simulink model "parent_model"  (R2024a)
settings: Solver=VariableStepAuto  StartTime=0.0  StopTime=50  RelTol=1e-3
libraries: aerolibutil x3, sharedtransform x1
settings Model: Creator=aryam  LastModifiedBy=ashis
settings RTWCC: GPUComputeCapability=3.5

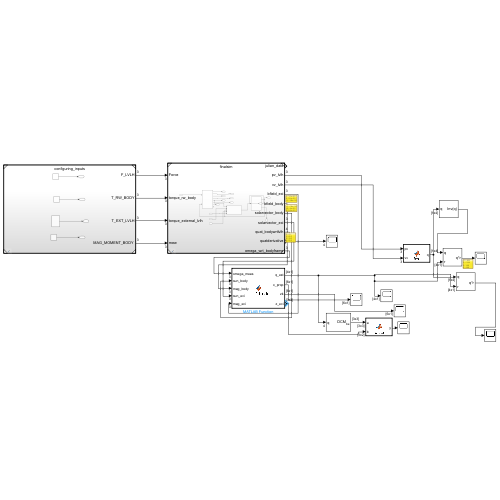
[thumbnail: Simulink's stored preview of the top-level diagram]
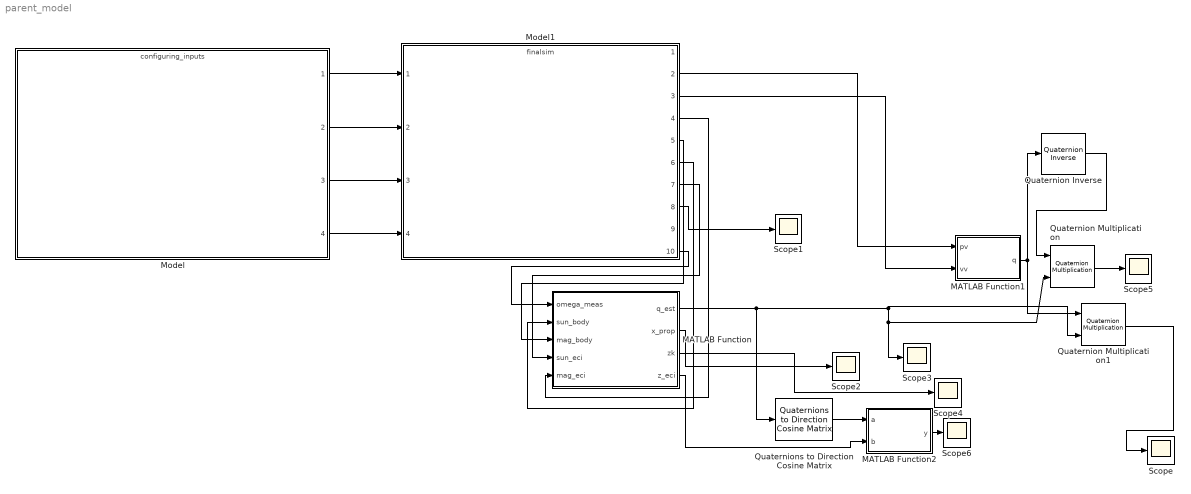
== system parent_model ==
  MATLAB Function : MATLAB Function  TreatAsAtomicUnit=on
  MATLAB Function1 : MATLAB Function  TreatAsAtomicUnit=on
  MATLAB Function2 : MATLAB Function  TreatAsAtomicUnit=on
  Model : ModelReference  ModelNameDialog=configuring_inputs.slx  SimulationMode=Normal  ModelReferenceVersion=2.0
  Model1 : ModelReference  ModelNameDialog=finalsim.slx  SimulationMode=Normal  ModelReferenceVersion=2.1
  Quaternion Inverse : aerolibutil/Quaternion Inverse
  Quaternion Multiplication : aerolibutil/Quaternion Multiplication
  Quaternion Multiplication1 : aerolibutil/Quaternion Multiplication
  Quaternions to Direction Cosine Matrix : sharedtransform/Quaternions to  Direction Cosine Matrix  aMode=aMode
      settings: LibrarySourceBlock=|
      | aerolibtransform2/Quaternions to
      | Direction Cosine Matrix
  Scope{,1..6} (7 alike) : Scope
  wires:
  Model/1 -> Model1/1
  Model/2 -> Model1/2
  Model/3 -> Model1/3
  Model/4 -> Model1/4
  Model1/7 -> MATLAB Function/4(sun_eci)
  Model1/10 -> MATLAB Function/1(omega_meas)
  Model1/5 -> MATLAB Function/3(mag_body)
  Model1/6 -> MATLAB Function/2(sun_body)
  Model1/4 -> MATLAB Function/5(mag_eci)
  Model1/8 -> Scope1/1
  MATLAB Function/2(x_prop) -> Scope2/1
  Model1/2 -> MATLAB Function1/1(pv)
  Model1/3 -> MATLAB Function1/2(vv)
  Quaternion Multiplication1/1 -> Scope/1
  MATLAB Function1/1(q) -> Quaternion Multiplication1/1, Quaternion Inverse/1
  MATLAB Function/1(q_est) -> Quaternions to Direction Cosine Matrix/1, Quaternion Multiplication/2, Scope3/1, Quaternion Multiplication1/2
  Quaternion Inverse/1 -> Quaternion Multiplication/1
  Quaternion Multiplication/1 -> Scope5/1
  Quaternions to Direction Cosine Matrix/1 -> MATLAB Function2/1(a)
  MATLAB Function/4(z_eci) -> MATLAB Function2/2(b)
  MATLAB Function/3(zk) -> Scope4/1
  MATLAB Function2/1(y) -> Scope6/1

== matlab function parent_model/MATLAB Function1 ==
  data: pv input; q output; vv input
function q = fcn(pv, vv)
    thirduv= -pv/norm(pv);
    seconduv=cross(thirduv, vv)/norm(cross(thirduv, vv));
    firstuv=cross(seconduv, thirduv ...
        );
    r=[firstuv, seconduv, thirduv];
    q=rotm2quat(r);
end

== matlab function parent_model/MATLAB Function ==
  settings: updateMethod=DISCRETE
  data: omega_meas input; q_est output; sun_body input; mag_body input; sun_eci input; mag_eci input; x_prop output; zk output; z_eci output
function [q_est, x_prop, zk, z_eci] = mekf_block(omega_meas, sun_body, mag_body, sun_eci, mag_eci)
    % Define the persistent MEKF object
    persistent mekf

    % Initialize the MEKF object on the first call
    if isempty(mekf)
        R_input = diag([0.01, 0.01, 0.01, 0.01, 0.01, 0.01]); % Example values
        P_start = eye(6); % Example values
        x_init = zeros(6, 1);
        dt = 0.1; % Example time step
        std_dev_process = [0.001, 0.001, 0.001, 0.01, 0.01, 0.01]; % Example values
        mekf = MEKF(R_input, P_start, x_init, dt, std_dev_process);
    end
    
    % Reset the MEKF object if required
    if norm(mekf.del_x(1:3)) > pi/12
        mekf = reset(mekf);
    end
    
    % Update the measurement
    zk = [sun_body; mag_body];
    mekf = measurement_update(mekf, zk, sun_eci, mag_eci);


    % Predict the state
    mekf = predict_state(mekf, omega_meas);
    
   
    % Output the estimated quaternion and propagated state
    q_est = mekf.q_prop;
    q_est_copy=q_est;
    q_est(1)=q_est_copy(4);
    q_est(2)=q_est_copy(1);
    q_est(3)=q_est_copy(2);
    q_est(4)=q_est_copy(3);
    x_prop = mekf.x_prop;
    z_eci = mag_eci;
end

== matlab function parent_model/MATLAB Function2 ==
  data: a input; y output; b input
function y = rotate(a, b)

y = a * b;
end
